simulink model "Linear_model"  (R2025a)
settings: Solver=ode4  StartTime=0.0  StopTime=1  FixedStep=0.0001  RelTol=1e-3
values from neighbouring files (symbols this model uses):
  A = [0 1; -(C/m) -(D/m)]    [Linear_model.m]    (also in TVRegDiff.m = @(v) cumsum(v))
  b = [0 ; K/m]    [Linear_model.m]
  c = [1 0]    [Linear_model.m]    (also in TVRegDiff.m = cumsum( n : -1 : 1 ).')
  d = 0    [Linear_model.m]
  Ts = 0.001    [Friction_line_identification.m]    (also in Linear_model.m; electromagnetic_actuator.m; nonlinear_model.m)
  x0 = [0 ; 0]    [Friction_line_identification.m]    (also in Linear_model.m; electromagnetic_actuator.m; nonlinear_model.m)
libraries: simulink x1
settings Model: Creator=Artur  LastModifiedBy=phill

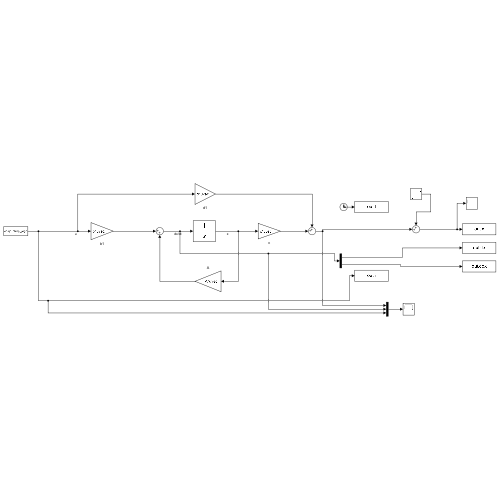
[thumbnail: Simulink's stored preview of the top-level diagram]
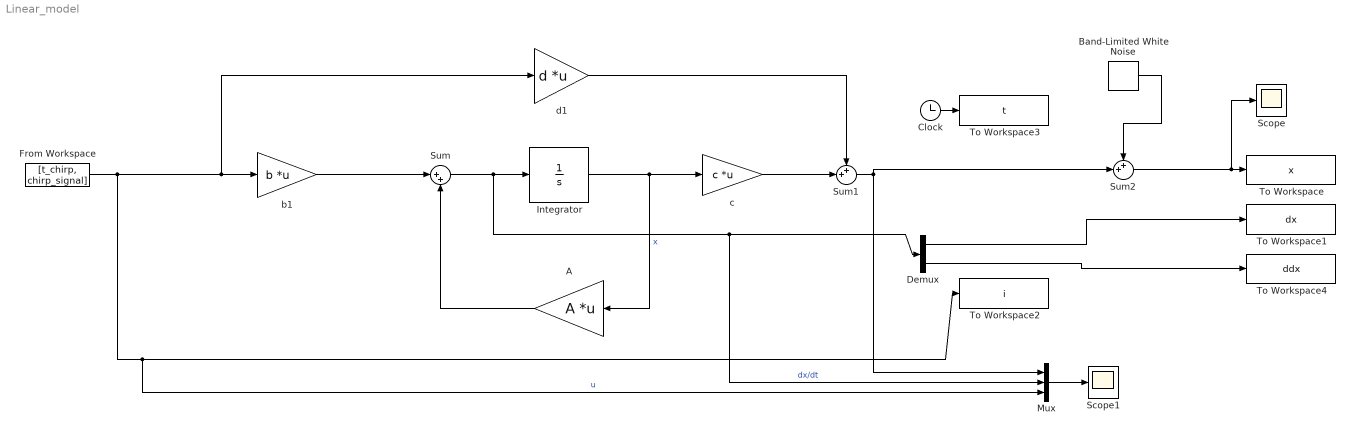
== system Linear_model ==
  A : Gain  Gain=A  Multiplication=Matrix(K*u) (u vector)
  Band-Limited White Noise : simulink/Sources/Band-Limited White Noise  Cov=[0.00000000001]  Ts=Ts  seed=[23341]
  Clock : Clock
  Demux : Demux  Outputs=2
  From Workspace : FromWorkspace  VariableName=[t_chirp, chirp_signal]
  Integrator : Integrator  InitialCondition=x0
  Mux : Mux  Inputs=3
  Scope : Scope
      settings: ActiveDisplayYMinimum=-0.001409054570019992  ActiveDisplayYMaximum=0.24899146493402396
  Scope1 : Scope
      settings: ActiveDisplayYMinimum=-7.3412624573538627  ActiveDisplayYMaximum=5.5321271901786586
  Sum : Sum  Inputs=|++
  Sum1 : Sum  Inputs=++|
  Sum2 : Sum  Inputs=++|
  To Workspace : ToWorkspace  VariableName=x  SampleTime=Ts
  To Workspace1 : ToWorkspace  VariableName=dx  SampleTime=Ts
  To Workspace2 : ToWorkspace  VariableName=i  SampleTime=Ts
  To Workspace3 : ToWorkspace  VariableName=t  SampleTime=Ts
  To Workspace4 : ToWorkspace  VariableName=ddx  SampleTime=Ts
  b1 : Gain  Gain=b  Multiplication=Matrix(K*u) (u vector)
  c : Gain  Gain=c  Multiplication=Matrix(K*u) (u vector)
  d1 : Gain  Gain=d  Multiplication=Matrix(K*u) (u vector)
  wires:
  d1/1 -> Sum1/1
  From Workspace/1 -> d1/1, b1/1, Mux/3, To Workspace2/1  "u"
  Sum/1 -> Mux/2, Demux/1, Integrator/1  "dx/dt"
  A/1 -> Sum/2
  c/1 -> Sum1/2
  b1/1 -> Sum/1
  Integrator/1 -> A/1, c/1  "x"
  Sum1/1 -> Mux/1, Sum2/2
  Clock/1 -> To Workspace3/1
  Mux/1 -> Scope1/1
  Sum2/1 -> Scope/1, To Workspace/1
  Band-Limited White Noise/1 -> Sum2/1
  Demux/1 -> To Workspace1/1
  Demux/2 -> To Workspace4/1
